simulink model "SPDCTL"  (R2022b)
settings: configuration reference "SharedConfig" (kept outside this file)
values from neighbouring files (symbols this model uses):
  DT_SPDCTL_C = 0.01    [SPDCTL.sldd]
  MotSpdRateLim_C = 1000.0    [SPDCTL.sldd]
  MotSpdReqMax_C = 1000.0    [SPDCTL.sldd]
  MotTqCmdSpdCtlDialEna_C = 0.0    [SPDCTL.sldd]
  MotTqCmdSpdCtlDialVal_C = 0.0    [SPDCTL.sldd]
  MotTqGainI_C = 0.0001    [SPDCTL.sldd]
  MotTqGainP_C = 0.0001    [SPDCTL.sldd]
undefined symbols (not defined in the file or in its folder): DiscIntNeverNeededParam, DRIVEMODE, slcm
libraries: simulink x4, BlockLibrary x1
Description:
  | Controls the motor speed in speed control mode.
settings Model: DataDictionary=SPDCTL.sldd  Creator=Kevin  LastModifiedBy=Max Kolesnikov
settings ConfigSetRef: SourceName=SharedConfig

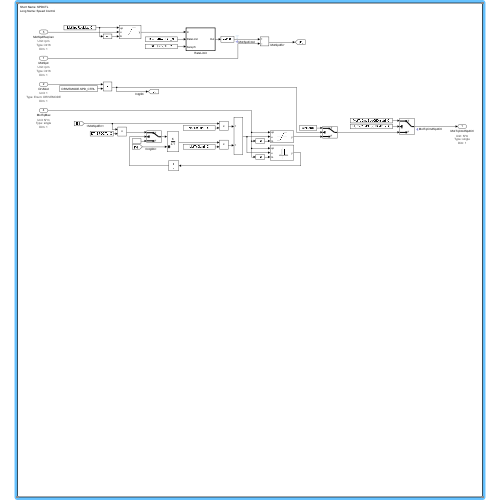
[thumbnail: Simulink's stored preview of the top-level diagram]
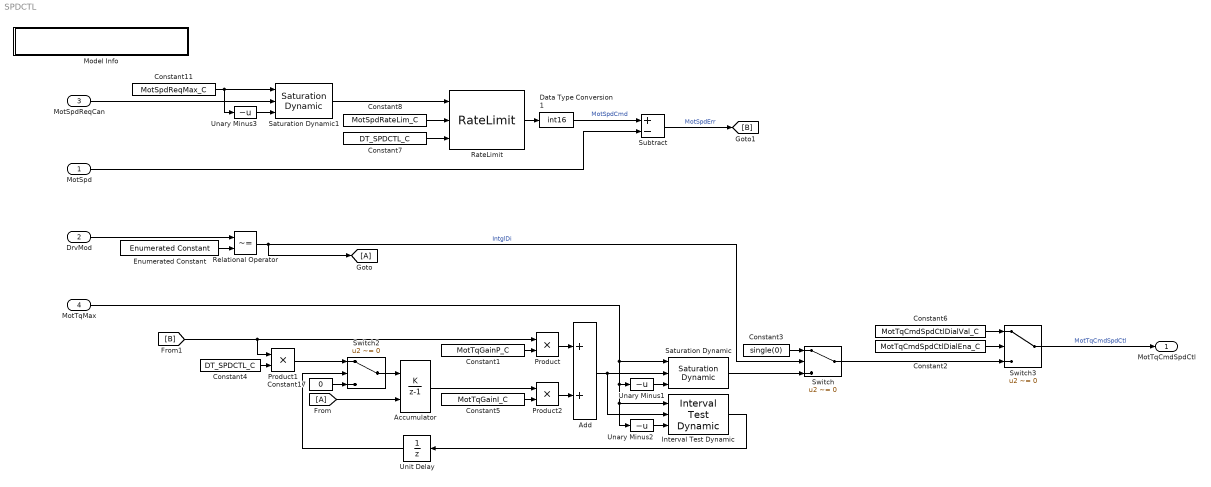
== system SPDCTL ==
  MotSpd : Inport  OutDataTypeStr=int16  Unit=rpm  PortDimensions=1
      settings: AttributesFormatString=|
      | Unit: %<Unit>
      | Type: %<OutDataTypeStr>
      | Dim: %<PortDimensions>
  DrvMod : Inport  Port=2  OutDataTypeStr=Enum: DRIVEMODE  Unit=1  PortDimensions=1
      settings: AttributesFormatString=|
      | Unit: %<Unit>
      | Type: %<OutDataTypeStr>
      | Dim: %<PortDimensions>
  MotSpdReqCan : Inport  Port=3  OutDataTypeStr=int16  Unit=rpm  PortDimensions=1
      settings: AttributesFormatString=|
      | Unit: %<Unit>
      | Type: %<OutDataTypeStr>
      | Dim: %<PortDimensions>
  MotTqMax : Inport  Port=4  OutDataTypeStr=single  Unit=N*m  PortDimensions=1
      settings: AttributesFormatString=|
      | Unit: %<Unit>
      | Type: %<OutDataTypeStr>
      | Dim: %<PortDimensions>
  Accumulator : DiscreteIntegrator  IntegratorMethod=Accumulation: Forward Euler  ExternalReset=level  SampleTime=-1  ICPrevOutput=DiscIntNeverNeededParam  ICPrevScaledInput=DiscIntNeverNeededParam
  Add : Sum
  Constant1 : Constant  Value=MotTqGainP_C
  Constant11 : Constant  Value=MotSpdReqMax_C
  Constant17 : Constant  Value=0  OutDataTypeStr=single
  Constant2 : Constant  Value=MotTqCmdSpdCtlDialEna_C
  Constant3 : Constant  Value=single(0)
  Constant4 : Constant  Value=DT_SPDCTL_C
  Constant5 : Constant  Value=MotTqGainI_C
  Constant6 : Constant  Value=MotTqCmdSpdCtlDialVal_C
  Constant7 : Constant  Value=DT_SPDCTL_C
  Constant8 : Constant  Value=MotSpdRateLim_C
  Data Type Conversion1 : DataTypeConversion  OutDataTypeStr=int16  SaturateOnIntegerOverflow=off  RndMeth=Floor
  Enumerated Constant : simulink/Sources/Enumerated Constant  OutDataTypeStr=Enum: DRIVEMODE  Value=DRIVEMODE.SPD_CTRL  SampleTime=inf
  From : From
  Goto : Goto
  Interval Test Dynamic : simulink/Logic and Bit Operations/Interval Test Dynamic  IntervalClosedRight=on  IntervalClosedLeft=on  OutDataTypeStr=boolean
  Model Info : Subsystem  LoadFcn=slcm LoadBlock;  InitFcn=slcm('UpdateAllCMBlocksInThisModelInit')  mask(CMBlock){Frame=off, DisplayStringWithTags=|, MaskDisplayString=Short Name: SPDCTL\nLong Name: Speed Control, HorizontalTextAlignment=Left, LeftAlignmentValue=0.02}
      mask DisplayStringWithTags=|
      | Short Name: %<ModelName>
      | Long Name: Speed Control
      mask prompts: Frame "Simulink:masks:Frame_MP"; DisplayStringWithTags "Simulink:masks:DisplayStringWithTags_MP"; MaskDisplayString "Simulink:masks:MaskDisplayString_MP"; HorizontalTextAlignment "Simulink:masks:HorizontalTextAlignment_MP"; LeftAlignmentValue "Simulink:masks:LeftAlignmentValue_MP"
      mask help: Simulink:masks:CMBlock_MD
      settings: CopyFcn=slcm CopyBlock;  DeleteFcn=slcm Cancel;  PostSaveFcn=slcm('UpdateAllCMBlocksInThisModel')  NameChangeFcn=slcm Rename;  OpenFcn=slcm
      mask Display: text(slResolve(LeftAlignmentValue, gcbh), 0.5, MaskDisplayString, 'HorizontalAlignment', HorizontalTextAlignment)
  Product : Product
  Product1 : Product
  Product2 : Product
  RateLimit : BlockLibrary/RateLimit  SystemSampleTime=-1  VariantActivationTime=update diagram  Latency=0  AutoFrameSizeCalculation=off
  Relational Operator : RelationalOperator  Operator=~=  OutDataTypeStr=boolean  RndMeth=Simplest  InputSameDT=off
  Saturation Dynamic : simulink/Discontinuities/Saturation Dynamic  OutMin=[]  OutMax=[]  OutDataTypeStr=Inherit: Same as second input  OutDataType=fixdt(1, 16)  OutScaling=2^-10  DoSatur=off
  Saturation Dynamic1 : simulink/Discontinuities/Saturation Dynamic  OutMin=[]  OutMax=[]  OutDataTypeStr=Inherit: Same as second input  OutDataType=fixdt(1, 16)  OutScaling=2^-10  DoSatur=off
  Subtract : Sum  Inputs=+-
  Switch : Switch  Criteria=u2 ~= 0  SaturateOnIntegerOverflow=off  InputSameDT=off
  Switch2 : Switch  Criteria=u2 ~= 0  SaturateOnIntegerOverflow=off  InputSameDT=off
  Switch3 : Switch  Criteria=u2 ~= 0  SaturateOnIntegerOverflow=off  InputSameDT=off
  Unary Minus1 : UnaryMinus
  Unary Minus2 : UnaryMinus
  Unary Minus3 : UnaryMinus
  Unit Delay : UnitDelay  SampleTime=-1  HasFrameUpgradeWarning=on
  MotTqCmdSpdCtl : Outport  OutDataTypeStr=single  Unit=N*m  PortDimensions=1
      settings: AttributesFormatString=|
      | Unit: %<Unit>
      | Type: %<OutDataTypeStr>
      | Dim: %<PortDimensions>
  wires:
  Constant1/1 -> Product/2
  Product/1 -> Add/1
  [B] -> Product/1, Product1/1
  Product1/1 -> Switch2/1
  Constant4/1 -> Product1/2
  DrvMod/1 -> Relational Operator/1
  Enumerated Constant/1 -> Relational Operator/2
  Switch3/1 -> MotTqCmdSpdCtl/1  "MotTqCmdSpdCtl"
  Constant3/1 -> Switch/1
  Constant8/1 -> RateLimit/2
  Constant7/1 -> RateLimit/3
  RateLimit/1 -> Data Type Conversion1/1
  Accumulator/1 -> Product2/1
  Constant5/1 -> Product2/2
  Product2/1 -> Add/2
  MotSpdReqCan/1 -> Saturation Dynamic1/2
  Add/1 -> Interval Test Dynamic/2, Saturation Dynamic/2
  MotTqMax/1 -> Saturation Dynamic/1, Unary Minus2/1, Interval Test Dynamic/1, Unary Minus1/1
  Saturation Dynamic/1 -> Switch/3
  Unary Minus1/1 -> Saturation Dynamic/3
  Unary Minus2/1 -> Interval Test Dynamic/3
  Interval Test Dynamic/1 -> Unit Delay/1
  Constant17/1 -> Switch2/3
  Unit Delay/1 -> Switch2/2
  Switch2/1 -> Accumulator/1
  Relational Operator/1 -> Switch/2, Goto/1  "IntglDi"
  From/1 -> Accumulator/2
  Data Type Conversion1/1 -> Subtract/1  "MotSpdCmd"
  MotSpd/1 -> Subtract/2
  Constant2/1 -> Switch3/2
  Constant6/1 -> Switch3/1
  Switch/1 -> Switch3/3
  Unary Minus3/1 -> Saturation Dynamic1/3
  Saturation Dynamic1/1 -> RateLimit/1
  Constant11/1 -> Saturation Dynamic1/1, Unary Minus3/1
  Subtract/1 -> [B]  "MotSpdErr"

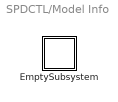
== system SPDCTL/Model Info ==
  EmptySubsystem : Subsystem

== system SPDCTL/Model Info/EmptySubsystem ==
